simulink model "jointTDtuning"  (R2021a)
settings: Solver=FixedStepDiscrete  StartTime=0.0  StopTime=Inf  FixedStep=0.001  RelTol=1e-3  EnableMultiTasking=on
PreLoadFcn:
  | set_param(gcs, 'RTWSystemTargetFile', 'franka_emika_panda.tlc');
  | % demos_common_configs();
values from neighbouring files (symbols this model uses):
  dof = 1    [jointTDtuning_init.m]
  init_delay = 10    [jointTDtuning_init.m]
  q_init = [65*pi/128, 59*pi/512, 0, -315 * pi/512, 0, 48*pi/64, 14*pi/64]    [jointTDtuning_init.m]
undefined symbols (not defined in the file or in its folder): DiscIntNeverNeededParam
libraries: spsSampleandHoldLib x12, franka_simulink_library x6, simulink x1, etargetslib x1, dspnetwork x1, dspsigops x1
settings Model: SimulationMode=external  ExtModeTrigDuration=10000  Creator=vasi_ko  LastModifiedBy=host
settings SolverCC: AlgebraicLoopSolver=TrustRegion
settings DataIOCC: LimitDataPoints=on  SaveFormat=Array  ReturnWorkspaceOutputs=off
settings OptimizationCC: EnhancedBackFolding=on  PassReuseOutputArgsThreshold=0  OptimizeBlockOrder=speed  DifferentSizesBufferReuse=on  OptimizationCustomize=off
settings DebuggingCC: SolverPrmCheckMsg=warning  ParameterTunabilityLossMsg=error  SFUnexpectedBacktrackingDiag=warning  SFNoUnconditionalDefaultTransitionDiag=warning  SFExecutionAtInitializationDiag=none  SFMachineParentedDataDiag=warning  ArithmeticOperatorsInVariantConditions=warning
settings HardwareCC: ProdBitPerLong=64  ProdHWDeviceType=Intel->x86-64 (Linux 64)
settings ModelReferenceCC: PropagateSignalLabelsOutOfModel=off
settings SFSimCC: SimUseLocalCustomCode=off  MATLABDynamicMemAlloc=off  CustomCodeUndefinedFunction=UseInterfaceOnly  SimTargetLang=C++
settings RTWCC: Description=Generic Real-Time Target  SystemTargetFile=franka_emika_panda.tlc  RTWVerbose=off  RTWUseLocalCustomCode=off  Toolchain=Franka Simulink | gmake (64-bit linux)  BuildConfiguration=Faster Runs  TargetLang=C++
settings CodeAppCC: ForceParamTrailComments=on  OperatorAnnotations=on
settings STFCustomTargetCC: TargetLangStandard=C99 (ISO)  ModelReferenceCompliant=off  MatFileLogging=on  SystemTargetFile=franka_emika_panda.tlc
settings GRTTargetCC: ModelReferenceCompliant=off  ParMdlRefBuildCompliant=off  CompOptLevelCompliant=off  ConcurrentExecutionCompliant=off  CombineOutputUpdateFcns=off  CPPClassGenCompliant=off  GRTInterface=on  ExtModeStaticAlloc=on  ExtModeTransport=1  ExtModeMexFile=ext_xcp  ExtModeIntrfLevel=Level2 - Open
settings ConfigComp: CovMetricSettings=dw  CovSaveCumulativeToWorkspaceVar=on  CovSaveSingleToWorkspaceVar=on  CovExternalEMLEnable=off  CovSFcnEnable=off

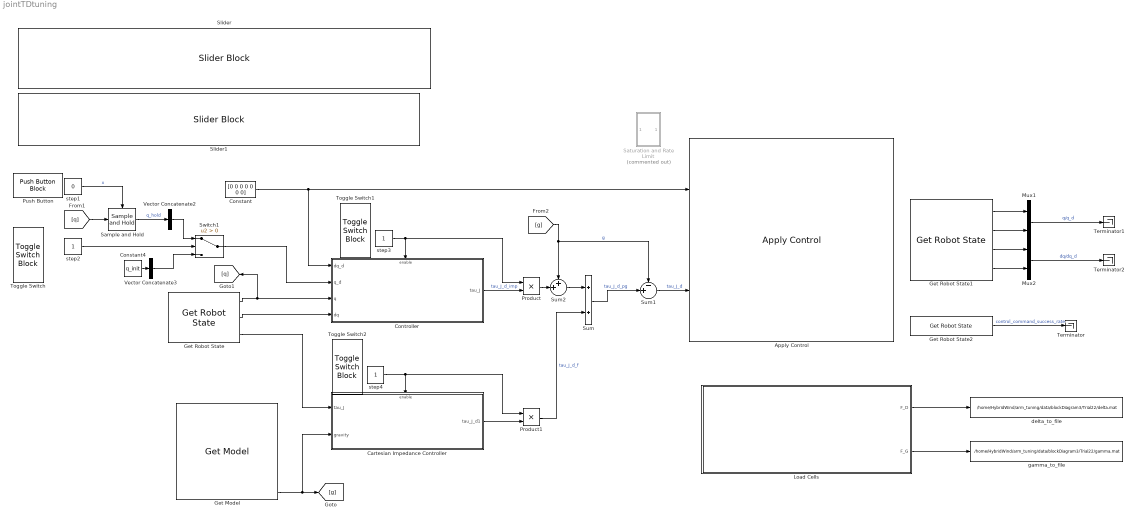
== system jointTDtuning ==
  Apply Control : franka_simulink_library/Apply Control  robot_ip=robot_ip  gripper_attached=off  control_mode=Torque Control - Joint Velocities  controller_choice=Joint Impedance Controller  elbow_control=on  collision_thresholds=100*ones(1,52)  joint_impedance=joint_impedance  cartesian_impedance=cartesian_impedance  load_inertia=load_inertia  EE_T_K=EE_T_K  init_joint_configuration_req=off  init_joint_configuration=q_init
      settings: SourceProductName=Franka Emika Simulink Support Package
  Cartesian Impedance Controller : Subsystem
      mask Display:
      | disp('{\bf\fontsize{18}Force Controller}', 'texmode','on');
      | %
      | % block_icon('Controller')
      | %
      | port_label('input',1,'tau_J');
      | port_label('output',1,'tau_J_d');
      | %port_label('output',2,'mass desired');
      | %port_label('output',3,'mass estimate');
  Constant : Constant  Value=[0 0 0 0 0 0 0]  VectorParams1D=off
  Constant4 : Constant  Value=q_init
  Controller : Subsystem
      mask Display:
      | % pos = get_param(gcb, 'Position');
      | 
      | disp('{\bf\fontsize{18}PD Controller}', 'texmode','on');
      | 
      | block_icon('Controller')
      | 
      | port_label('output',1,'tau_J_d');
      | 
      | port_label('input',2,'q_d');
      | port_label('input',1,'dq_d');
      | port_label('input',3,'q');
      | port_label('input',4,'dq');
  Get Model : franka_simulink_library/Get Model  robot_ip=robot_ip
      settings: SourceProductName=Franka Emika Simulink Support Package
  Get Robot State : franka_simulink_library/Get Robot State  robot_ip=robot_ip  signals_requested='q dq tau_J'
      settings: SourceProductName=Franka Emika Simulink Support Package
  Get Robot State1 : franka_simulink_library/Get Robot State  robot_ip=robot_ip  signals_requested='q q_d dq dq_d'
      settings: SourceProductName=Franka Emika Simulink Support Package
  Get Robot State2 : franka_simulink_library/Get Robot State  robot_ip=robot_ip  signals_requested='control_command_success_rate'
      settings: SourceProductName=Franka Emika Simulink Support Package
  Load Cells : Subsystem
  Mux1 : Mux  Inputs=2
  Mux2 : Mux  Inputs=2
  Product : Product
  Product1 : Product
  Push Button : PushButtonBlock
  Sample and Hold : dspsigops/Sample and Hold  trig=Rising edge  initCond=q_init  latchinput=off
  Saturation and Rate Limit : Subsystem  Commented=on
  Slider : SliderBlock  ScaleMax=3  TickInterval=0.25
  Slider1 : SliderBlock  ScaleMax=2
  Sum : Sum
  Sum1 : Sum  Inputs=-+|
  Sum2 : Sum  Inputs=++|
  Switch1 : Switch  Criteria=u2 > Threshold
  Terminator : Terminator
  Terminator1 : Terminator
  Terminator2 : Terminator
  Toggle Switch : ToggleSwitchBlock
      settings: Values={{'Off', 'On'}, [0 1]}
  Toggle Switch1 : ToggleSwitchBlock
      settings: Values={{'Off', 'On'}, [0 1]}
  Toggle Switch2 : ToggleSwitchBlock
      settings: Values={{'Off', 'On'}, [0 1]}
  Vector Concatenate2 : Concatenate  NumInputs=1
  Vector Concatenate3 : Concatenate  NumInputs=1
  delta_to_file : ToFile  Filename=/home/HybridWind/arm_tuning/data/blockDiagram3/Trial22/delta.mat  MatrixName=delta
  gamma_to_file : ToFile  Filename=/home/HybridWind/arm_tuning/data/blockDiagram3/Trial22/gamma.mat  MatrixName=gamma
  step1 : Constant  Value=0
  step2 : Constant
  step3 : Constant
  step4 : Constant
  wires:
  Switch1/1 -> Controller/2(q_d)
  [q] -> Sample and Hold/1
  Sum/1 -> Sum1/2  "tau_J_d_pg"
  Vector Concatenate2/1 -> Switch1/1
  Constant4/1 -> Vector Concatenate3/1
  Get Robot State/3 -> Cartesian Impedance Controller/1(tau_J)
  Get Model/6 -> [g], Cartesian Impedance Controller/2(gravity)
  Load Cells/1(F_D) -> delta_to_file/1
  Cartesian Impedance Controller/1(tau_J_d1) -> Product1/2
  Get Robot State1/4 -> Mux2/2
  step2/1 -> Switch1/2
  Get Robot State1/3 -> Mux2/1
  Get Robot State2/1 -> Terminator/1  "control_command_success_rate"
  Product/1 -> Sum2/2
  Mux1/1 -> Terminator1/1  "q/q_d"
  Sample and Hold/1 -> Vector Concatenate2/1  "q_hold"
  Get Robot State1/1 -> Mux1/1
  Get Robot State1/2 -> Mux1/2
  Vector Concatenate3/1 -> Switch1/3
  Constant/1 -> Apply Control/1, Controller/1(dq_d)
  step4/1 -> Product1/1, Cartesian Impedance Controller/Enable
  Get Robot State/2 -> Controller/4(dq)
  Get Robot State/1 -> [q], Controller/3(q)
  Sum1/1 -> Apply Control/2  "tau_J_d"
  Controller/1(tau_J) -> Product/2  "tau_J_d_imp"
  step1/1 -> Sample and Hold/Trigger  "x"
  step3/1 -> Product/1, Controller/Enable
  Mux2/1 -> Terminator2/1  "dq/dq_d"
  Load Cells/2(F_G) -> gamma_to_file/1
  Product1/1 -> Sum/2  "tau_J_d_f"
  [g] -> Sum1/1, Sum2/1  "g"
  Sum2/1 -> Sum/1

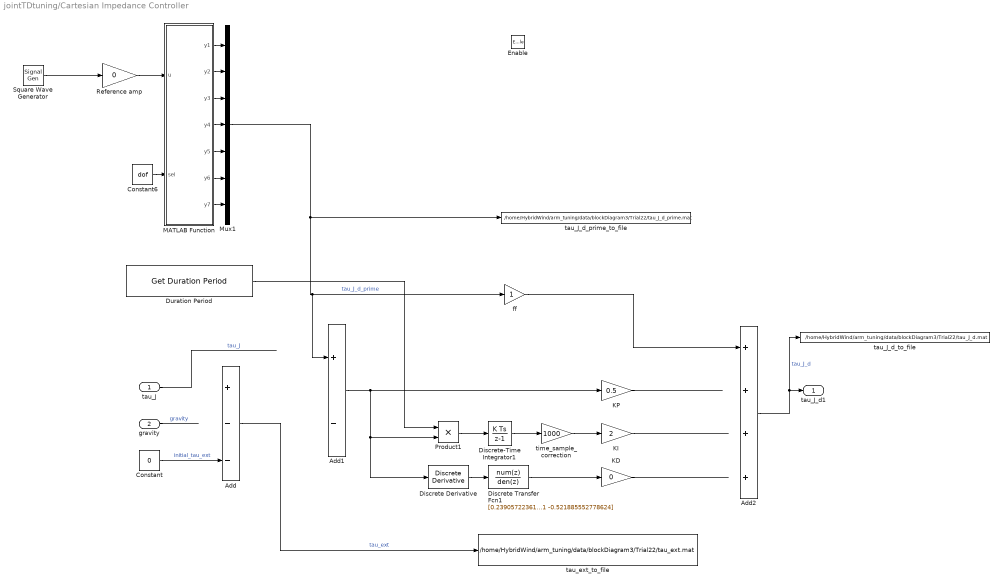
== system jointTDtuning/Cartesian Impedance Controller ==
  tau_J : Inport
  gravity : Inport  Port=2
  Enable : EnablePort  StatesWhenEnabling=reset
  Add : Sum  Inputs=+--
  Add1 : Sum  Inputs=+-
  Add2 : Sum  Inputs=++++
  Constant : Constant  Value=0
  Constant6 : Constant  Value=dof
  Discrete Transfer Fcn1 : DiscreteTransferFcn  Numerator=[0.239057223610688 0.239057223610688]  Denominator=[1 -0.521885552778624]
  Discrete Derivative : simulink/Discrete/Discrete Derivative  gainval=1.0  ICPrevScaledInput=0.0  OutMin=[]  OutMax=[]  OutDataType=fixdt(1, 16)  OutScaling=2^-10  DoSatur=off
  Discrete-Time Integrator1 : DiscreteIntegrator  SampleTime=0.001  ICPrevOutput=DiscIntNeverNeededParam  ICPrevScaledInput=DiscIntNeverNeededParam
  Duration Period : franka_simulink_library/Get Duration Period  robot_ip=robot_ip
      settings: SourceProductName=Franka Emika Simulink Support Package
  KD : Gain  Gain=0
  KI : Gain  Gain=2
  KP : Gain  Gain=0.5
  MATLAB Function : MATLAB Function  TreatAsAtomicUnit=on
  Mux1 : Mux  Inputs=7
  Product1 : Product
  Reference amp : Gain  Gain=0
  Square Wave Generator : SignalGenerator  WaveForm=square  Amplitude=5
  ff : Gain
  tau_J_d_prime_to_file : ToFile  Filename=/home/HybridWind/arm_tuning/data/blockDiagram3/Trial22/tau_J_d_prime.mat  MatrixName=tau_J_d_prime
  tau_J_d_to_file : ToFile  Filename=/home/HybridWind/arm_tuning/data/blockDiagram3/Trial22/tau_J_d.mat  MatrixName=tau_J_d
  tau_ext_to_file : ToFile  Filename=/home/HybridWind/arm_tuning/data/blockDiagram3/Trial22/tau_ext.mat  MatrixName=tau_ext
  time_sample_correction : Gain  Gain=1000
  tau_J_d1 : Outport  InitialOutput=[0 0 0 0 0 0 0]  VectorParamsAs1DForOutWhenUnconnected=off
  wires:
  Add1/1 -> Discrete Derivative/1, Product1/2, KP/1
  Constant/1 -> Add/3  "initial_tau_ext"
  MATLAB Function/1(y1) -> Mux1/1
  MATLAB Function/4(y4) -> Mux1/4
  Reference amp/1 -> MATLAB Function/1(u)
  Add2/1 -> tau_J_d_to_file/1, tau_J_d1/1  "tau_J_d"
  Discrete Transfer Fcn1/1 -> KD/1
  MATLAB Function/6(y6) -> Mux1/6
  KD/1 -> ?
  MATLAB Function/2(y2) -> Mux1/2
  MATLAB Function/5(y5) -> Mux1/5
  Square Wave Generator/1 -> Reference amp/1
  Add/1 -> tau_ext_to_file/1  "tau_ext"
  KP/1 -> ?
  tau_J/1 -> ?  "tau_J"
  MATLAB Function/3(y3) -> Mux1/3
  Constant6/1 -> MATLAB Function/2(sel)
  gravity/1 -> ?  "gravity"
  MATLAB Function/7(y7) -> Mux1/7
  Mux1/1 -> tau_J_d_prime_to_file/1, Add1/1, ff/1  "tau_J_d_prime"
  ff/1 -> Add2/1
  KI/1 -> ?
  Duration Period/1 -> Product1/1
  Discrete Derivative/1 -> Discrete Transfer Fcn1/1
  Product1/1 -> Discrete-Time Integrator1/1
  Discrete-Time Integrator1/1 -> time_sample_correction/1
  time_sample_correction/1 -> KI/1

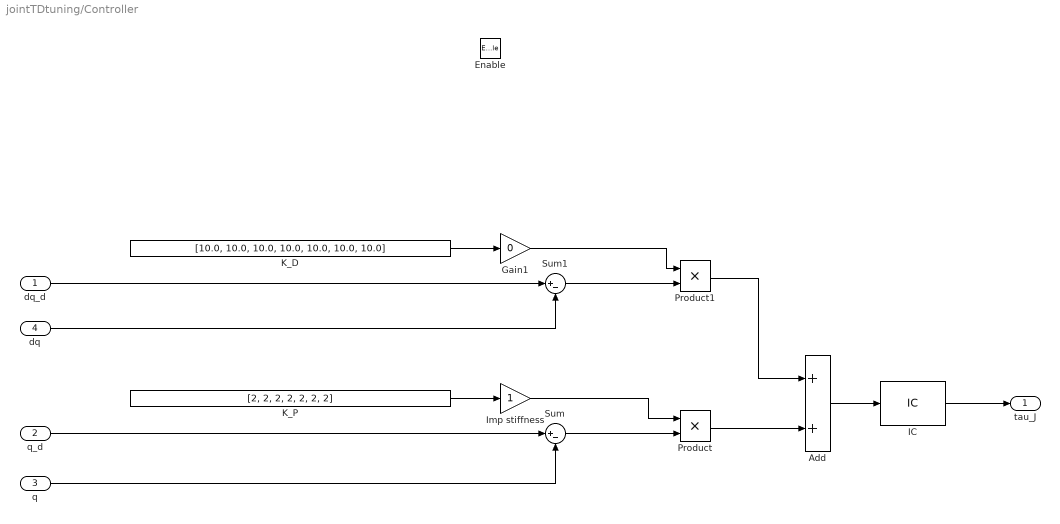
== system jointTDtuning/Controller ==
  dq_d : Inport
  q_d : Inport  Port=2
  q : Inport  Port=3
  dq : Inport  Port=4
  Enable : EnablePort  StatesWhenEnabling=reset
  Add : Sum
  Gain1 : Gain  Gain=0
  IC : InitialCondition  Value=zeros(1,7)
  Imp stiffness : Gain
  K_D : Constant  Value=[10.0, 10.0, 10.0, 10.0, 10.0, 10.0, 10.0]  VectorParams1D=off  SampleTime=-1
  K_P : Constant  Value=[2, 2, 2, 2, 2, 2, 2]  VectorParams1D=off  SampleTime=-1
  Product : Product
  Product1 : Product
  Sum : Sum  Inputs=|+-
  Sum1 : Sum  Inputs=|+-
  tau_J : Outport  VectorParamsAs1DForOutWhenUnconnected=off
  wires:
  Add/1 -> IC/1
  Sum1/1 -> Product1/2
  dq/1 -> Sum1/2
  q_d/1 -> Sum/1
  dq_d/1 -> Sum1/1
  Product1/1 -> Add/1
  Product/1 -> Add/2
  K_D/1 -> Gain1/1
  K_P/1 -> Imp stiffness/1
  Sum/1 -> Product/2
  q/1 -> Sum/2
  Imp stiffness/1 -> Product/1
  Gain1/1 -> Product1/1
  IC/1 -> tau_J/1

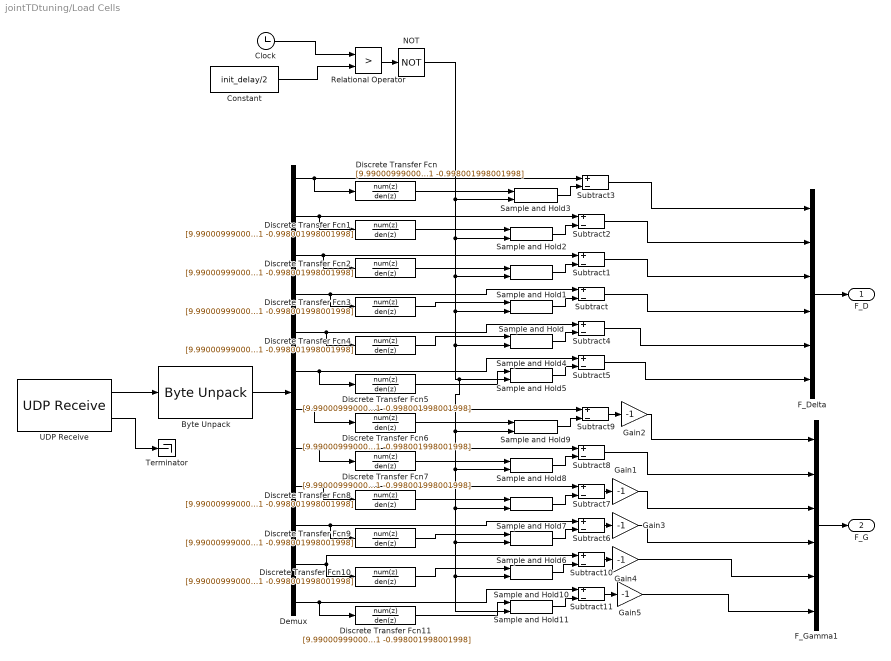
== system jointTDtuning/Load Cells ==
  Byte Unpack : etargetslib/Byte Unpack  dimensions={[12]}  datatypes={'double'}  byteAlign=1
  Clock : Clock
  Constant : Constant  Value=init_delay/2
  Demux : Demux  Outputs=12
  Discrete Transfer Fcn{,1..11} (12 alike) : DiscreteTransferFcn  Numerator=[9.990009990009990e-04 9.990009990009990e-04]  Denominator=[1 -0.998001998001998]
  F_Delta : Mux  Inputs=6
  F_Gamma1 : Mux  Inputs=6
  Gain{1..5} (5 alike) : Gain  Gain=-1
  NOT : Logic  Operator=NOT  IconShape=distinctive  AllPortsSameDT=off  OutDataTypeStr=boolean
  Relational Operator : RelationalOperator  Operator=>  OutDataTypeStr=boolean  RndMeth=Simplest
  Sample and Hold{,1..11} (12 alike) : spsSampleandHoldLib/Sample and Hold  ic=0  Ts=0
      settings: SourceProductBaseCode=PS
  Subtract{,1..11} (12 alike) : Sum  Inputs=+-
  Terminator : Terminator
  UDP Receive : dspnetwork/UDP Receive  localURL='0.0.0.0'  localPort=8002  remoteURL='10.10.10.15'  remotePort=-1  recvBufferSize=8192  dims=96  signalDatatype=uint8  isComplex=off  isVarSize=off  showBlockingTime=on  blockingTime=inf  sampletime=0.001  blockPlatform=HOST
  F_D : Outport
  F_G : Outport  Port=2
  wires:
  UDP Receive/1 -> Byte Unpack/1
  Constant/1 -> Relational Operator/2
  Relational Operator/1 -> NOT/1
  Sample and Hold/1 -> Subtract/2
  UDP Receive/2 -> Terminator/1
  Demux/4 -> Discrete Transfer Fcn3/1, Subtract/1
  Clock/1 -> Relational Operator/1
  Byte Unpack/1 -> Demux/1
  Demux/3 -> Discrete Transfer Fcn2/1, Subtract1/1
  Sample and Hold1/1 -> Subtract1/2
  Subtract1/1 -> F_Delta/3
  Subtract2/1 -> F_Delta/2
  Sample and Hold2/1 -> Subtract2/2
  Demux/2 -> Discrete Transfer Fcn1/1, Subtract2/1
  Sample and Hold3/1 -> Subtract3/2
  Subtract4/1 -> F_Delta/5
  Sample and Hold4/1 -> Subtract4/2
  Demux/5 -> Discrete Transfer Fcn4/1, Subtract4/1
  Demux/6 -> Discrete Transfer Fcn5/1, Subtract5/1
  Sample and Hold5/1 -> Subtract5/2
  Subtract5/1 -> F_Delta/6
  Subtract3/1 -> F_Delta/1
  Subtract/1 -> F_Delta/4
  F_Delta/1 -> F_D/1
  Demux/1 -> Discrete Transfer Fcn/1, Subtract3/1
  Discrete Transfer Fcn/1 -> Sample and Hold3/1
  Discrete Transfer Fcn1/1 -> Sample and Hold2/1
  Discrete Transfer Fcn2/1 -> Sample and Hold1/1
  Discrete Transfer Fcn3/1 -> Sample and Hold/1
  Discrete Transfer Fcn4/1 -> Sample and Hold4/1
  Discrete Transfer Fcn5/1 -> Sample and Hold5/1
  Discrete Transfer Fcn11/1 -> Sample and Hold11/1
  Discrete Transfer Fcn10/1 -> Sample and Hold10/1
  Discrete Transfer Fcn9/1 -> Sample and Hold6/1
  Discrete Transfer Fcn8/1 -> Sample and Hold7/1
  Discrete Transfer Fcn7/1 -> Sample and Hold8/1
  Discrete Transfer Fcn6/1 -> Sample and Hold9/1
  Demux/7 -> Subtract9/1, Discrete Transfer Fcn6/1
  F_Gamma1/1 -> F_G/1
  Gain3/1 -> F_Gamma1/4
  Gain2/1 -> F_Gamma1/1
  Subtract11/1 -> Gain5/1
  Sample and Hold11/1 -> Subtract11/2
  NOT/1 -> Sample and Hold3/2, Sample and Hold2/2, Sample and Hold1/2, Sample and Hold6/2, Sample and Hold10/2, Sample and Hold11/2, Sample and Hold7/2, Sample and Hold8/2, Sample and Hold9/2, Sample and Hold5/2, Sample and Hold4/2, Sample and Hold/2
  Demux/12 -> Subtract11/1, Discrete Transfer Fcn11/1
  Demux/11 -> Subtract10/1, Discrete Transfer Fcn10/1
  Sample and Hold10/1 -> Subtract10/2
  Gain4/1 -> F_Gamma1/5
  Subtract9/1 -> Gain2/1
  Sample and Hold9/1 -> Subtract9/2
  Demux/8 -> Subtract8/1, Discrete Transfer Fcn7/1
  Sample and Hold8/1 -> Subtract8/2
  Subtract8/1 -> F_Gamma1/2
  Gain1/1 -> F_Gamma1/3
  Sample and Hold7/1 -> Subtract7/2
  Demux/9 -> Subtract7/1, Discrete Transfer Fcn8/1
  Demux/10 -> Subtract6/1, Discrete Transfer Fcn9/1
  Sample and Hold6/1 -> Subtract6/2
  Subtract6/1 -> Gain3/1
  Subtract7/1 -> Gain1/1
  Subtract10/1 -> Gain4/1
  Gain5/1 -> F_Gamma1/6

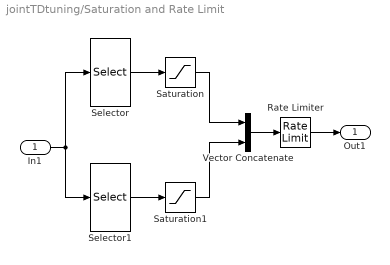
== system jointTDtuning/Saturation and Rate Limit ==
  In1 : Inport
  Rate Limiter : RateLimiter  RisingSlewLimit=1000  FallingSlewLimit=-1000  SampleTimeMode=inherited
  Saturation : Saturate  UpperLimit=87  LowerLimit=-87
  Saturation1 : Saturate  UpperLimit=12  LowerLimit=-12
  Selector : Selector  InputPortWidth=7  IndexOptions=Index vector (dialog)  Indices=[1 2 3 4]  OutputSizes=1
  Selector1 : Selector  InputPortWidth=7  IndexOptions=Index vector (dialog)  Indices=[5 6 7]  OutputSizes=1
  Vector Concatenate : Concatenate
  Out1 : Outport
  wires:
  Saturation1/1 -> Vector Concatenate/2
  Vector Concatenate/1 -> Rate Limiter/1
  Saturation/1 -> Vector Concatenate/1
  Rate Limiter/1 -> Out1/1
  Selector1/1 -> Saturation1/1
  Selector/1 -> Saturation/1
  In1/1 -> Selector1/1, Selector/1

== matlab function jointTDtuning/Cartesian Impedance Controller/MATLAB Function ==
  data: u input; y1 output; sel input; y2 output; y3 output; y4 output; y5 output; y6 output; y7 output
function [y1, y2, y3, y4, y5, y6, y7] = fcn(u, sel)

y1 = 0;
y2 = 0;
y3 = 0;
y4 = 0;
y5 = 0;
y6 = 0;
y7 = 0;

switch sel
    case 1
        y1 = u;
    case 2
        y2 = u;
    case 3
        y3 = u;
    case 4
        y4 = u;
    case 5
        y5 = u;
    case 6
        y6 = u;
    case 7
        y7 = u;
    otherwise
        y1 = 0;
end
